simulink model "hybrid"  (Simulink 8.5)
settings: Solver=ode5  StartTime=0.0  StopTime=3  RelTol=1e-3
settings Model: Creator=syaghoub  LastModifiedBy=adokhanc
settings DataIOCC: InitialState=X0  LimitDataPoints=off  SaveFinalState=on  SignalLoggingSaveFormat=Dataset  SaveState=on
settings OptimizationCC: ExpressionDepthLimit=128
settings DebuggingCC: UnderspecifiedInitializationDetection=Simplified  MergeDetectMultiDrivingBlocksExec=error  FcnCallInpInsideContextMsg=EnableAllAsError  StateNameClashWarn=none  InitInArrayFormatMsg=none
settings HardwareCC: ProdBitPerPointer=64  ProdLargestAtomicFloat=Float  ProdIntDivRoundTo=Zero  ProdEndianess=LittleEndian  ProdHWDeviceType=Specified
settings ModelReferenceCC: PropagateSignalLabelsOutOfModel=on
settings GRTTargetCC: CombineOutputUpdateFcns=on  GRTInterface=off

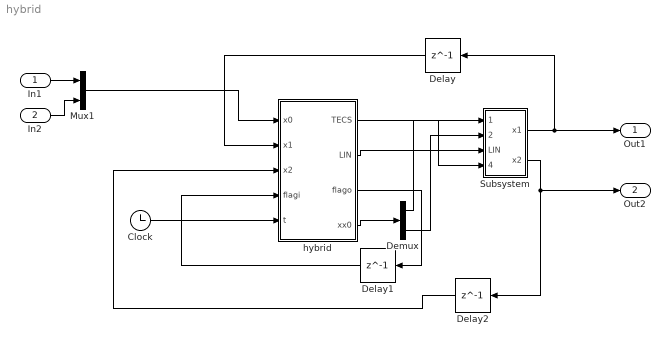
== system hybrid ==
  In1 : Inport
  In2 : Inport  Port=2
  Clock : Clock
  Delay : Delay  DelayLength=1  InitialCondition=0
  Delay1 : Delay  DelayLength=1  InitialCondition=0
  Delay2 : Delay  DelayLength=1  InitialCondition=0
  Demux : Demux  Outputs=2
  Mux1 : Mux  Inputs=2
  Subsystem : Subsystem
  hybrid : MATLAB Function  TreatAsAtomicUnit=on
  Out1 : Outport
  Out2 : Outport  Port=2
  wires:
  hybrid/1(TECS) -> Subsystem/4(TECS)
  hybrid/2(LIN) -> Subsystem/3(LIN)
  Subsystem/2(x2) -> Delay2/1, Out2/1
  Subsystem/1(x1) -> Delay/1, Out1/1
  Clock/1 -> hybrid/5(t)
  hybrid/3(flago) -> Delay1/1
  Delay1/1 -> hybrid/4(flagi)
  Mux1/1 -> hybrid/1(x0)
  hybrid/4(xx0) -> Demux/1
  Demux/1 -> Subsystem/1(x10)
  Demux/2 -> Subsystem/2(x20)
  Delay2/1 -> hybrid/3(x2)
  Delay/1 -> hybrid/2(x1)
  In1/1 -> Mux1/1
  In2/1 -> Mux1/2

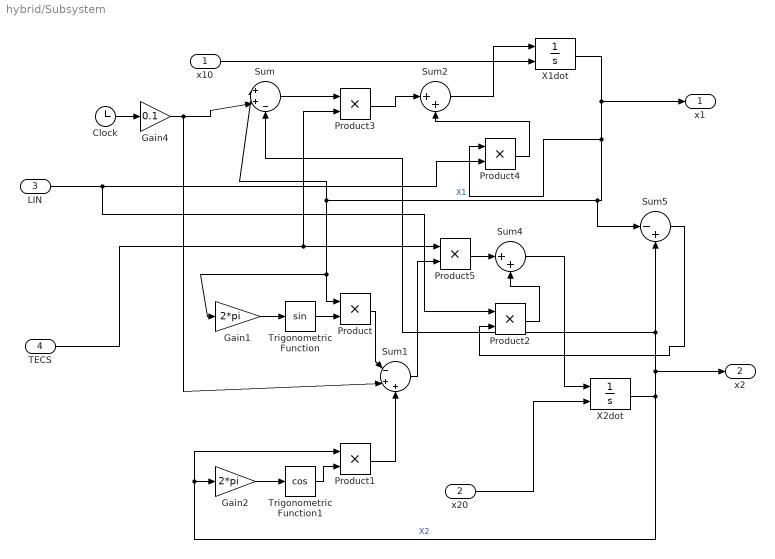
== system hybrid/Subsystem ==
  x10 : Inport
  x20 : Inport  Port=2
  LIN : Inport  Port=3
  TECS : Inport  Port=4
  Clock : Clock
  Gain1 : Gain  Gain=2*pi
  Gain2 : Gain  Gain=2*pi
  Gain4 : Gain  Gain=0.1
  Product{,1..5} (6 alike) : Product
  Sum : Sum  Inputs=|++-
  Sum1 : Sum  Inputs=|-++
  Sum2 : Sum  Inputs=|++
  Sum4 : Sum  Inputs=|++
  Sum5 : Sum  Inputs=|-+
  Trigonometric Function : Trigonometry
  Trigonometric Function1 : Trigonometry  Operator=cos
  X1dot : Integrator  InitialConditionSource=external  InitialCondition=0.5
  X2dot : Integrator  InitialConditionSource=external  InitialCondition=0.5
  x1 : Outport
  x2 : Outport  Port=2
  wires:
  X1dot/1 -> Product4/1, Sum5/1, Sum/1, Product/1, Gain1/1, x1/1  "X1"
  Trigonometric Function/1 -> Product/2
  X2dot/1 -> x2/1, Sum5/2, Sum/3, Gain2/1, Product1/1  "X2"
  Gain2/1 -> Trigonometric Function1/1
  Trigonometric Function1/1 -> Product1/2
  Gain1/1 -> Trigonometric Function/1
  Product1/1 -> Sum1/3
  Product/1 -> Sum1/1
  x20/1 -> X2dot/2
  Gain4/1 -> Sum1/2, Sum/2
  x10/1 -> X1dot/2
  Clock/1 -> Gain4/1
  Product4/1 -> Sum2/2
  Sum2/1 -> X1dot/1
  Sum1/1 -> Product5/2
  Product5/1 -> Sum4/1
  Product2/1 -> Sum4/2
  Sum4/1 -> X2dot/1
  Sum5/1 -> Product2/2
  TECS/1 -> Product3/2, Product5/1
  LIN/1 -> Product2/1, Product4/2
  Sum/1 -> Product3/1
  Product3/1 -> Sum2/1

== matlab function hybrid ==
  data: x0 input double; x1 input double; x2 input double; TECS output double; LIN output double; flago output double; flagi input double; t input double; xx0 output double
function [TECS,LIN,flago,xx0] = fcn(x0,x1,x2,flagi,t)
XU=[0.85,.95;
    0.85,0.95];
if 0.02>=t
    if ~ ( ( x0(1)>XU(1,1) && x0(1)<XU(1,2) && x0(2)>XU(2,1) && x0(2)<XU(2,2) ) )
        TECS=1;
        LIN=0;
        flago=0;
    else 
        LIN=1;
        TECS=0;
        flago=1;
    end  
    xx0=x0;
else
    if ~ ( ( x1>XU(1,1) && x1<XU(1,2) && x2>XU(2,1) && x2<XU(2,2) ) || 0.5<=flagi )
        TECS=1;
        LIN=0;
        flago=flagi;
    else 
        LIN=1;
        TECS=0;
        flago=1;
    end
    xx0=x0;
end

end
% function [dy] = TECSODE(t,x)
% %% Flow_TECS
% dy = [x(1)-x(2) + 0.1*t;
%     x(2)*cos(2*pi*x(2)) - x(1)*sin(2*pi*x(1))+0.1*t];
% end
% function [dy] = LINODE(t,x)
% %% Flow_Lin
% dy = [x(1);
%     -x(2)+ x(1)];
% end
